simulink model "model"  (R2020b)
settings: Solver=VariableStepAuto  StartTime=0.0  StopTime=100  RelTol=1e-3
settings Model: Creator=SAGAR  LastModifiedBy=SAGAR

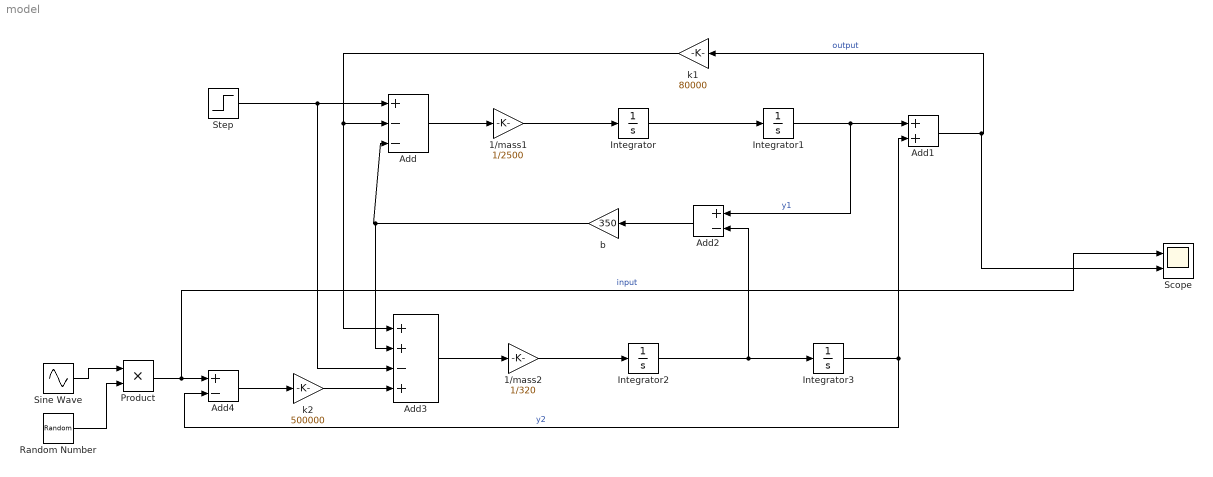
== system model ==
  1/mass1 : Gain  Gain=1/2500
  1/mass2 : Gain  Gain=1/320
  Add : Sum  Inputs=+--
  Add1 : Sum
  Add2 : Sum  Inputs=+-
  Add3 : Sum  Inputs=++-+
  Add4 : Sum  Inputs=+-
  Integrator{,1..3} (4 alike) : Integrator
  Product : Product
  Random Number : RandomNumber  SampleTime=0.1
  Scope : Scope  NumInputPorts=2
  Sine Wave : Sin  SampleTime=0
  Step : Step  SampleTime=0
  b : Gain  Gain=350
  k1 : Gain  Gain=80000
  k2 : Gain  Gain=500000
  wires:
  Integrator/1 -> Integrator1/1
  Add/1 -> 1/mass1/1
  1/mass1/1 -> Integrator/1
  Integrator1/1 -> Add2/1, Add1/1  "y1"
  Add1/1 -> Scope/2, k1/1  "output"
  k1/1 -> Add3/1, Add/2
  Add2/1 -> b/1
  b/1 -> Add3/2, Add/3
  Add3/1 -> 1/mass2/1
  1/mass2/1 -> Integrator2/1
  Integrator2/1 -> Add2/2, Integrator3/1
  Integrator3/1 -> Add4/2, Add1/2  "y2"
  k2/1 -> Add3/4
  Step/1 -> Add3/3, Add/1
  Add4/1 -> k2/1
  Sine Wave/1 -> Product/1
  Random Number/1 -> Product/2
  Product/1 -> Scope/1, Add4/1  "input"
